simulink model "lab_4"  (R2021b)
settings: Solver=VariableStepAuto  StartTime=0.0  StopTime=t  RelTol=1e-3
values from neighbouring files (symbols this model uses):
  adaptive = 1    [env_lab_4.m]
  Am = A - b*K    [env_lab_4.m]
  Bm = b    [env_lab_4.m]
  ga = diag([10 10 10 10])    [env_lab_4.m]
  gb = 10    [env_lab_4.m]
  J1 = 0.05    [env_lab_4.m]
  J2 = J2_init    (= 0.1)    [env_lab_4.m]
  K = acker(A, b, P)    [env_lab_4.m]
  ke = 1    [env_lab_4.m]
  km = 1    [env_lab_4.m]
  Kn = Kn_init    [env_lab_4.m]
  L = 0.01    [env_lab_4.m]
  modal = i    [env_lab_4.m]
  P = [-5 -5 -5 -5]    [env_lab_4.m]
  p = p_init    (= 0.0333333333333)    [env_lab_4.m]
  pulse_period = 12    [env_lab_4.m]
  R = 2    [env_lab_4.m]
settings Model: Creator=Данил  LastModifiedBy=79159
settings DebuggingCC: UnconnectedInputMsg=none  UnconnectedOutputMsg=none  UnconnectedLineMsg=none
settings RTWCC: DLArmComputeVersion=20.02.1

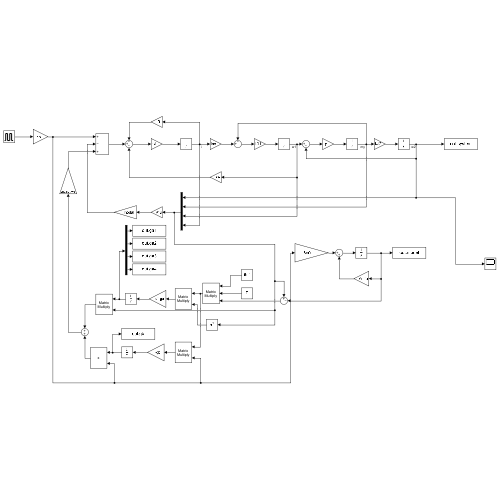
[thumbnail: Simulink's stored preview of the top-level diagram]
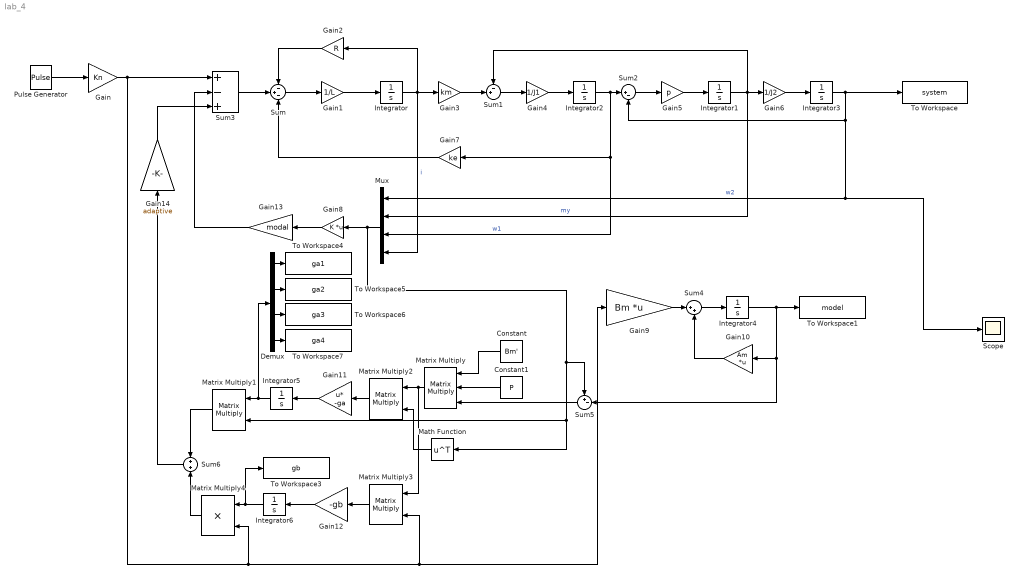
== system lab_4 ==
  Constant : Constant  Value=Bm'  VectorParams1D=off
  Constant1 : Constant  Value=P  VectorParams1D=off
  Demux : Demux
  Gain : Gain  Gain=Kn
  Gain1 : Gain  Gain=1/L
  Gain10 : Gain  Gain=Am  Multiplication=Matrix(K*u)
  Gain11 : Gain  Gain=-ga  Multiplication=Matrix(u*K)
  Gain12 : Gain  Gain=-gb
  Gain13 : Gain  Gain=modal
  Gain14 : Gain  Gain=adaptive
  Gain2 : Gain  Gain=R
  Gain3 : Gain  Gain=km
  Gain4 : Gain  Gain=1/J1
  Gain5 : Gain  Gain=p
  Gain6 : Gain  Gain=1/J2
  Gain7 : Gain  Gain=ke
  Gain8 : Gain  Gain=K  Multiplication=Matrix(K*u)
  Gain9 : Gain  Gain=Bm  Multiplication=Matrix(K*u)
  Integrator{,1..6} (7 alike) : Integrator
  Math Function : Math  Operator=transpose  SaturateOnIntegerOverflow=on
  Matrix Multiply : Product  Inputs=3  Multiplication=Matrix(*)
  Matrix Multiply1 : Product  Multiplication=Matrix(*)
  Matrix Multiply2 : Product  Multiplication=Matrix(*)
  Matrix Multiply3 : Product  Multiplication=Matrix(*)
  Matrix Multiply4 : Product
  Mux : Mux
  Pulse Generator : DiscretePulseGenerator  PulseType=Time based  Period=pulse_period  PulseWidth=50
  Scope : Scope
  Sum : Sum  Inputs=-+-
  Sum1 : Sum  Inputs=-+|
  Sum2 : Sum  Inputs=|+-
  Sum3 : Sum  Inputs=+-+
  Sum4 : Sum  Inputs=|++
  Sum5 : Sum  Inputs=+-|
  Sum6 : Sum
  To Workspace : ToWorkspace  VariableName=system  SaveFormat=Timeseries  SampleTime=-1
  To Workspace1 : ToWorkspace  VariableName=model  SaveFormat=Timeseries  SampleTime=-1
  To Workspace3 : ToWorkspace  VariableName=gb  SaveFormat=Timeseries  SampleTime=-1
  To Workspace4 : ToWorkspace  VariableName=ga1  SaveFormat=Timeseries  SampleTime=-1
  To Workspace5 : ToWorkspace  VariableName=ga2  SaveFormat=Timeseries  SampleTime=-1
  To Workspace6 : ToWorkspace  VariableName=ga3  SaveFormat=Timeseries  SampleTime=-1
  To Workspace7 : ToWorkspace  VariableName=ga4  SaveFormat=Timeseries  SampleTime=-1
  wires:
  Sum/1 -> Gain1/1
  Gain1/1 -> Integrator/1
  Integrator/1 -> Mux/4, Gain2/1, Gain3/1  "i"
  Gain2/1 -> Sum/1
  Gain3/1 -> Sum1/2
  Sum1/1 -> Gain4/1
  Gain4/1 -> Integrator2/1
  Integrator2/1 -> Mux/3, Gain7/1, Sum2/1  "w1"
  Sum2/1 -> Gain5/1
  Gain5/1 -> Integrator1/1
  Gain6/1 -> Integrator3/1
  Integrator1/1 -> Mux/2, Gain6/1, Sum1/1  "my"
  Integrator3/1 -> To Workspace/1, Scope/1, Mux/1, Sum2/2  "w2"
  Gain7/1 -> Sum/3
  Mux/1 -> Gain8/1, Sum5/1, Math Function/1, Matrix Multiply1/2
  Sum3/1 -> Sum/2
  Gain/1 -> Sum3/1, Gain9/1, Matrix Multiply3/2, Matrix Multiply4/2
  Gain9/1 -> Sum4/1
  Sum4/1 -> Integrator4/1
  Integrator4/1 -> To Workspace1/1, Sum5/2, Gain10/1
  Gain10/1 -> Sum4/2
  Constant/1 -> Matrix Multiply/1
  Constant1/1 -> Matrix Multiply/2
  Sum5/1 -> Matrix Multiply/3
  Gain11/1 -> Integrator5/1
  Integrator5/1 -> Demux/1, Matrix Multiply1/1
  Matrix Multiply/1 -> Matrix Multiply3/1, Matrix Multiply2/1
  Matrix Multiply2/1 -> Gain11/1
  Math Function/1 -> Matrix Multiply2/2
  Matrix Multiply3/1 -> Gain12/1
  Gain12/1 -> Integrator6/1
  Integrator6/1 -> To Workspace3/1, Matrix Multiply4/1
  Matrix Multiply1/1 -> Sum6/1
  Matrix Multiply4/1 -> Sum6/2
  Pulse Generator/1 -> Gain/1
  Gain13/1 -> Sum3/2
  Gain8/1 -> Gain13/1
  Sum6/1 -> Gain14/1
  Gain14/1 -> Sum3/3
  Demux/1 -> To Workspace4/1
  Demux/2 -> To Workspace5/1
  Demux/3 -> To Workspace6/1
  Demux/4 -> To Workspace7/1
